simulink model "controller_linear"  (R2023a)
settings: Solver=VariableStepAuto  StartTime=0.0  StopTime=10.0  RelTol=1e-3
values from neighbouring files (symbols this model uses):
  den = [1, 0, -30.17, 0, 0]    [Grp43_part2_code.m]
  denC = [1, q0]    [Grp43_part2_code.m]
  num1 = [a0, a1]    [Grp43_part2_code.m]
  num2 = [p0, p1]    [Grp43_part2_code.m]
  numX = [0.4167, 0, -12.41]    [Grp43_part2_code.m]
  numY = [-0.15, 0, 0]    [Grp43_part2_code.m]
settings Model: Creator=Anirvan Krishna  LastModifiedBy=Anirvan Krishna

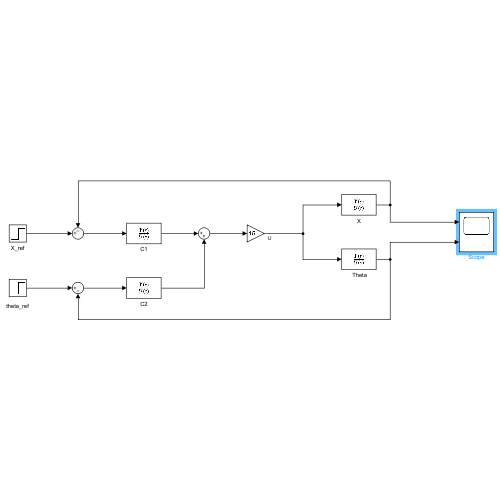
[thumbnail: Simulink's stored preview of the top-level diagram]
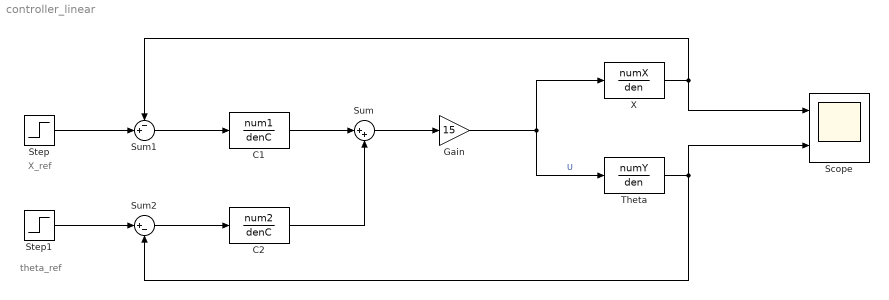
== system controller_linear ==
  note: X_ref
  note: theta_ref
  " Theta" : TransferFcn  Numerator=numY  Denominator=den  ContinuousStateAttributes='g2'
  C1 : TransferFcn  Numerator=num1  Denominator=denC  ContinuousStateAttributes='c1'
  C2 : TransferFcn  Numerator=num2  Denominator=denC  ContinuousStateAttributes='c2'
  Gain : Gain  Gain=15
  Scope : Scope  NumInputPorts=2
  Step : Step  Time=0.1  SampleTime=0
  Step1 : Step  Time=0.1  SampleTime=0
  Sum : Sum  Inputs=|++
  Sum1 : Sum  Inputs=-+|
  Sum2 : Sum  Inputs=|+-
  X : TransferFcn  Numerator=numX  Denominator=den  ContinuousStateAttributes='g1'
  wires:
  Gain/1 -> " Theta"/1, X/1  "U"
  C1/1 -> Sum/1
  C2/1 -> Sum/2
  Sum/1 -> Gain/1
  X/1 -> Sum1/1, Scope/1
  " Theta"/1 -> Sum2/2, Scope/2
  Sum2/1 -> C2/1
  Sum1/1 -> C1/1
  Step/1 -> Sum1/2
  Step1/1 -> Sum2/1
